simulink model "SPGF_FSK_0000_R2020b"  (R2020b)
settings: Solver=ode4  StartTime=0.0  StopTime=1.4  FixedStep=50e-6/50  RelTol=1e-3  EnableMultiTasking=on
undefined symbols (not defined in the file): D11, Delta
libraries: powerlib x2546, powerlib_meascontrol x183, simulink x24
(part 2 of 34)

== system SPGF_FSK_0000_R2020b/K4 ==
  fault : Subsystem  mask{FaultA=on, FaultB=off, FaultC=off, FaultResistance=0.0001, GroundResistance=1e-03, SnubberResistance=1e6, SnubberCapacitance=inf, TransitionTimes=[0.2 0.8], TheoryOfArc=None, ArcingVoltage=6000, TypeOfPause=None, NoiseSampleTime=0.04, NoiseSeed=23345, PulsePeriod=0.2, PulseWidth=20, PhaseDelay=0.2, SwitchTimes=[0.2 0.225 0.5 0.6], LimitArcNum=off, ArcingNumber=1, AddTimeDelay=off, TimeDelay=[0 0.1 0.2 ]}
      mask prompts: FaultA "Phase A Fault"; FaultB "Phase B Fault"; FaultC "Phase C Fault"; FaultResistance "Fault resistance Ron (ohms) :"; GroundResistance "Ground resistance Rg (ohms) :"; SnubberResistance "Snubbers resistance Rp (ohms) :"; SnubberCapacitance "Snubbers capacitance Cp (F) :"; TransitionTimes "Transition times (s) :"; TheoryOfArc "Theory of the arcing ground"; ArcingVoltage "Voltage of the arcing (V) :"; TypeOfPause "Add pause in the arcing ground"; NoiseSampleTime "Sample time of white noise (s) :"; NoiseSeed "Seed of white noise"; PulsePeriod "Period of pulses (s) :"; PulseWidth "Width of pulse (% of period) :"; PhaseDelay "Phase delay (sec) :"; SwitchTimes "Switch times (sec) [1,0,1,0...] :"; LimitArcNum "Limit number of arcing [N] :"; ArcingNumber "Number of uprising arcing"; AddTimeDelay "Add time delay :"; TimeDelay "Time delay between arc (sec) [1xN] :"
      mask init: same as SPGF_FSK_0000_R2020b/K1/fault
      settings: CloseFcn=|
      | en = get_param(gcb,'MaskEnables');
      | set_param(gcb,'MaskEnables',en)
      | clear enab en;
      settings: MoveFcn=|
      | en = get_param(gcb,'MaskEnables');
      | set_param(gcb,'MaskEnables',en)
      | clear enab en;
      mask Callback FaultA:
      | enab = get_param(gcb,'FaultA');
      | en = get_param(gcb,'MaskEnables');
      | % Set the 'MaskVisililities' property for each parameters
      | if strcmp(enab,'on')
      |     en{2}='off';
      |     en{3}='off';
      | % set_param(gcb,'MaskVisibilities',{'on','on','on','on','on','on','on','on','on','off','on','',''});
      | else
      |     en{2}='on';
      |     en{3}='on';
      | % set_param(gcb,'MaskVisibilities',{'on','on','on','on','on','on','on','on','on','on','on','',''});
      | end
      | set_param(gcb,'MaskEnables',en)
      | clear enab en;
      mask Callback FaultB:
      | enab = get_param(gcb,'FaultB');
      | en = get_param(gcb,'MaskEnables');
      | % Set the 'MaskVisililities' property for each parameters
      | if strcmp(enab,'on')
      |     en{1}='off';
      |     en{3}='off';
      | % set_param(gcb,'MaskVisibilities',{'on','on','on','on','on','on','on','on','on','off','on','',''});
      | else
      |     en{1}='on';
      |     en{3}='on';
      | % set_param(gcb,'MaskVisibilities',{'on','on','on','on','on','on','on','on','on','on','on','',''});
      | end
      | set_param(gcb,'MaskEnables',en)
      | clear enab en;
      mask Callback FaultC:
      | enab = get_param(gcb,'FaultC');
      | en = get_param(gcb,'MaskEnables');
      | % Set the 'MaskVisililities' property for each parameters
      | if strcmp(enab,'on')
      |     en{1}='off';
      |     en{2}='off';
      | % set_param(gcb,'MaskVisibilities',{'on','on','on','on','on','on','on','on','on','off','on','',''});
      | else
      |     en{1}='on';
      |     en{2}='on';
      | % set_param(gcb,'MaskVisibilities',{'on','on','on','on','on','on','on','on','on','on','on','',''});
      | end
      | set_param(gcb,'MaskEnables',en)
      | clear enab en;
      mask TypeOptions TheoryOfArc: None | Petersen | Peters & Slepian
      mask Callback TheoryOfArc:
      | enab = get_param(gcb,'TheoryOfArc');
      | en = get_param(gcb,'MaskEnables');
      | % Set the 'MaskVisililities' property for each parameters
      | if strcmp(enab,'None')
      |     en{10}='off';
      | % set_param(gcb,'MaskVisibilities',{'on','on','on','on','on','on','on','on','on','off','on','',''});
      | else
      |     en{10}='on';
      | % set_param(gcb,'MaskVisibilities',{'on','on','on','on','on','on','on','on','on','on','on','',''});
      | end
      | set_param(gcb,'MaskEnables',en)
      | clear enab en;
      mask TypeOptions TypeOfPause: None | White Noise | Pulse Generator | Time Dependent Pulses
      mask Callback TypeOfPause:
      | enab = get_param(gcb,'TypeOfPause');
      | en = get_param(gcb,'MaskVisibilities');
      | % Set the 'MaskVisibilities' property for each parameters
      | if strcmp(enab,'None')
      |     en{12} = 'off';
      |     en{13} = 'off';
      |     en{14} = 'off';
      |     en{15} = 'off';
      |     en{16} = 'off';
      |     en{17} = 'off';
      | % set_param(gcb,'MaskEnables',{'on','on','on','on','on','on','on','on','on','on','on','on','on'});
      | elseif strcmp(enab,'White Noise')
      |     en{12} = 'on';
      |     en{13} = 'on';
      |     en{14} = 'off';
      |     en{15} = 'off';
      |     en{16} = 'off';
      |     en{17} = 'off';
      | elseif strcmp(enab,'Pulse Generator')
      |     en{12} = 'off';
      |     en{13} = 'off';
      |     en{14} = 'on';
      |     en{15} = 'on';
      |     en{16} = 'on';
      |     en{17} = 'off';
      | else
      |     en{12} = 'off';
      |     en{13} = 'off';
      |     en{14} = 'off';
      |     en{15} = 'off';
      |     en{16} = 'off';
      |     en{17} = 'on';
      | % set_param(gcb,'Maskenables',{'on','on','on','on','on','on','on','on','on','on','on','off','off'});
      | end
      | set_param(gcb,'MaskVisibilities',en);
      | clear enab en;
      mask Callback LimitArcNum:
      | enab = get_param(gcb,'LimitArcNum');
      | en = get_param(gcb,'MaskVisibilities');
      | % Set the 'MaskVisibilities' property for each parameters
      | if strcmp(enab,'on')
      |     en{19} = 'on';
      |     en{20} = 'on';
      |     en{21} = 'on';
      | else
      |     en{19} = 'off';
      |     en{20} = 'off';
      |     set_param(gcb,'AddTimeDelay','off');
      |     en{21} = 'off';
      | % set_param(gcb,'Maskenables',{'on','on','on','on','on','on','on','on','on','on','on','off','off'});
      | end
      | set_param(gcb,'MaskVisibilities',en);
      | clear enab en;
      mask Callback AddTimeDelay:
      | enab = get_param(gcb,'AddTimeDelay');
      | en = get_param(gcb,'MaskVisibilities');
      | % Set the 'MaskVisibilities' property for each parameters
      | if strcmp(enab,'on')
      |     en{21} = 'on';
      | else
      |     en{21} = 'off';
      | % set_param(gcb,'Maskenables',{'on','on','on','on','on','on','on','on','on','on','on','off','off'});
      | end
      | set_param(gcb,'MaskVisibilities',en);
      | clear enab en;
      mask Display:
      | % port_label('input',1,'Iabc');
      | 
      | port_label('lconn',1,'A');
      | port_label('lconn',2,'B');
      | port_label('lconn',3,'C');
      | 
      | disp('   ПДЗ    ');
  meas : Subsystem
  A : PMIOPort  Side=Left
  B : PMIOPort  Port=2  Side=Left
  C : PMIOPort  Port=3  Side=Left
  connections:
  meas/LConn3 -- C/RConn1
  meas/LConn1 -- A/RConn1
  meas/LConn2 -- B/RConn1
  fault/LConn3 -- meas/RConn3
  fault/LConn2 -- meas/RConn2
  fault/LConn1 -- meas/RConn1

== system SPGF_FSK_0000_R2020b/K5 ==
  fault : Subsystem  mask{FaultA=off, FaultB=off, FaultC=off, FaultResistance=0.0001, GroundResistance=1e-03, SnubberResistance=1e6, SnubberCapacitance=inf, TransitionTimes=[1.2 1.8], TheoryOfArc=Peters & Slepian, ArcingVoltage=6000, TypeOfPause=None, NoiseSampleTime=0.04, NoiseSeed=23345, PulsePeriod=0.2, PulseWidth=20, PhaseDelay=0, SwitchTimes=[1 1.01 1.2 1.4], LimitArcNum=on, ArcingNumber=1, AddTimeDelay=off, TimeDelay=[0 0.1 0.2 ]}
      mask prompts: FaultA "Phase A Fault"; FaultB "Phase B Fault"; FaultC "Phase C Fault"; FaultResistance "Fault resistance Ron (ohms) :"; GroundResistance "Ground resistance Rg (ohms) :"; SnubberResistance "Snubbers resistance Rp (ohms) :"; SnubberCapacitance "Snubbers capacitance Cp (F) :"; TransitionTimes "Transition times (s) :"; TheoryOfArc "Theory of the arcing ground"; ArcingVoltage "Voltage of the arcing (V) :"; TypeOfPause "Add pause in the arcing ground"; NoiseSampleTime "Sample time of white noise (s) :"; NoiseSeed "Seed of white noise"; PulsePeriod "Period of pulses (s) :"; PulseWidth "Width of pulse (% of period) :"; PhaseDelay "Phase delay (sec) :"; SwitchTimes "Switch times (sec) [1,0,1,0...] :"; LimitArcNum "Limit number of arcing [N] :"; ArcingNumber "Number of uprising arcing"; AddTimeDelay "Add time delay :"; TimeDelay "Time delay between arc (sec) [1xN] :"
      mask init: same as SPGF_FSK_0000_R2020b/K1/fault
      settings: CloseFcn=|
      | en = get_param(gcb,'MaskEnables');
      | set_param(gcb,'MaskEnables',en)
      | clear enab en;
      settings: MoveFcn=|
      | en = get_param(gcb,'MaskEnables');
      | set_param(gcb,'MaskEnables',en)
      | clear enab en;
      mask Callback FaultA:
      | enab = get_param(gcb,'FaultA');
      | en = get_param(gcb,'MaskEnables');
      | % Set the 'MaskVisililities' property for each parameters
      | if strcmp(enab,'on')
      |     en{2}='off';
      |     en{3}='off';
      | % set_param(gcb,'MaskVisibilities',{'on','on','on','on','on','on','on','on','on','off','on','',''});
      | else
      |     en{2}='on';
      |     en{3}='on';
      | % set_param(gcb,'MaskVisibilities',{'on','on','on','on','on','on','on','on','on','on','on','',''});
      | end
      | set_param(gcb,'MaskEnables',en)
      | clear enab en;
      mask Callback FaultB:
      | enab = get_param(gcb,'FaultB');
      | en = get_param(gcb,'MaskEnables');
      | % Set the 'MaskVisililities' property for each parameters
      | if strcmp(enab,'on')
      |     en{1}='off';
      |     en{3}='off';
      | % set_param(gcb,'MaskVisibilities',{'on','on','on','on','on','on','on','on','on','off','on','',''});
      | else
      |     en{1}='on';
      |     en{3}='on';
      | % set_param(gcb,'MaskVisibilities',{'on','on','on','on','on','on','on','on','on','on','on','',''});
      | end
      | set_param(gcb,'MaskEnables',en)
      | clear enab en;
      mask Callback FaultC:
      | enab = get_param(gcb,'FaultC');
      | en = get_param(gcb,'MaskEnables');
      | % Set the 'MaskVisililities' property for each parameters
      | if strcmp(enab,'on')
      |     en{1}='off';
      |     en{2}='off';
      | % set_param(gcb,'MaskVisibilities',{'on','on','on','on','on','on','on','on','on','off','on','',''});
      | else
      |     en{1}='on';
      |     en{2}='on';
      | % set_param(gcb,'MaskVisibilities',{'on','on','on','on','on','on','on','on','on','on','on','',''});
      | end
      | set_param(gcb,'MaskEnables',en)
      | clear enab en;
      mask TypeOptions TheoryOfArc: None | Petersen | Peters & Slepian
      mask Callback TheoryOfArc:
      | enab = get_param(gcb,'TheoryOfArc');
      | en = get_param(gcb,'MaskEnables');
      | % Set the 'MaskVisililities' property for each parameters
      | if strcmp(enab,'None')
      |     en{10}='off';
      | % set_param(gcb,'MaskVisibilities',{'on','on','on','on','on','on','on','on','on','off','on','',''});
      | else
      |     en{10}='on';
      | % set_param(gcb,'MaskVisibilities',{'on','on','on','on','on','on','on','on','on','on','on','',''});
      | end
      | set_param(gcb,'MaskEnables',en)
      | clear enab en;
      mask TypeOptions TypeOfPause: None | White Noise | Pulse Generator | Time Dependent Pulses
      mask Callback TypeOfPause:
      | enab = get_param(gcb,'TypeOfPause');
      | en = get_param(gcb,'MaskVisibilities');
      | % Set the 'MaskVisibilities' property for each parameters
      | if strcmp(enab,'None')
      |     en{12} = 'off';
      |     en{13} = 'off';
      |     en{14} = 'off';
      |     en{15} = 'off';
      |     en{16} = 'off';
      |     en{17} = 'off';
      | % set_param(gcb,'MaskEnables',{'on','on','on','on','on','on','on','on','on','on','on','on','on'});
      | elseif strcmp(enab,'White Noise')
      |     en{12} = 'on';
      |     en{13} = 'on';
      |     en{14} = 'off';
      |     en{15} = 'off';
      |     en{16} = 'off';
      |     en{17} = 'off';
      | elseif strcmp(enab,'Pulse Generator')
      |     en{12} = 'off';
      |     en{13} = 'off';
      |     en{14} = 'on';
      |     en{15} = 'on';
      |     en{16} = 'on';
      |     en{17} = 'off';
      | else
      |     en{12} = 'off';
      |     en{13} = 'off';
      |     en{14} = 'off';
      |     en{15} = 'off';
      |     en{16} = 'off';
      |     en{17} = 'on';
      | % set_param(gcb,'Maskenables',{'on','on','on','on','on','on','on','on','on','on','on','off','off'});
      | end
      | set_param(gcb,'MaskVisibilities',en);
      | clear enab en;
      mask Callback LimitArcNum:
      | enab = get_param(gcb,'LimitArcNum');
      | en = get_param(gcb,'MaskVisibilities');
      | % Set the 'MaskVisibilities' property for each parameters
      | if strcmp(enab,'on')
      |     en{19} = 'on';
      |     en{20} = 'on';
      |     en{21} = 'on';
      | else
      |     en{19} = 'off';
      |     en{20} = 'off';
      |     set_param(gcb,'AddTimeDelay','off');
      |     en{21} = 'off';
      | % set_param(gcb,'Maskenables',{'on','on','on','on','on','on','on','on','on','on','on','off','off'});
      | end
      | set_param(gcb,'MaskVisibilities',en);
      | clear enab en;
      mask Callback AddTimeDelay:
      | enab = get_param(gcb,'AddTimeDelay');
      | en = get_param(gcb,'MaskVisibilities');
      | % Set the 'MaskVisibilities' property for each parameters
      | if strcmp(enab,'on')
      |     en{21} = 'on';
      | else
      |     en{21} = 'off';
      | % set_param(gcb,'Maskenables',{'on','on','on','on','on','on','on','on','on','on','on','off','off'});
      | end
      | set_param(gcb,'MaskVisibilities',en);
      | clear enab en;
      mask Display:
      | % port_label('input',1,'Iabc');
      | 
      | port_label('lconn',1,'A');
      | port_label('lconn',2,'B');
      | port_label('lconn',3,'C');
      | 
      | disp('   ПДЗ    ');
  meas : Subsystem
  A : PMIOPort  Side=Left
  B : PMIOPort  Port=2  Side=Left
  C : PMIOPort  Port=3  Side=Left
  connections:
  fault/LConn1 -- meas/RConn1
  fault/LConn2 -- meas/RConn2
  fault/LConn3 -- meas/RConn3
  meas/LConn2 -- B/RConn1
  meas/LConn1 -- A/RConn1
  meas/LConn3 -- C/RConn1

== system SPGF_FSK_0000_R2020b/K6 ==
  fault : Subsystem  mask{FaultA=on, FaultB=off, FaultC=off, FaultResistance=0.0001, GroundResistance=1e-03, SnubberResistance=1e6, SnubberCapacitance=inf, TransitionTimes=[0.2 0.8], TheoryOfArc=None, ArcingVoltage=6000, TypeOfPause=None, NoiseSampleTime=0.04, NoiseSeed=23345, PulsePeriod=0.2, PulseWidth=20, PhaseDelay=0, SwitchTimes=[1 1.01 1.2 1.4], LimitArcNum=off, ArcingNumber=1, AddTimeDelay=off, TimeDelay=[0 0.1 0.2 ]}
      mask prompts: FaultA "Phase A Fault"; FaultB "Phase B Fault"; FaultC "Phase C Fault"; FaultResistance "Fault resistance Ron (ohms) :"; GroundResistance "Ground resistance Rg (ohms) :"; SnubberResistance "Snubbers resistance Rp (ohms) :"; SnubberCapacitance "Snubbers capacitance Cp (F) :"; TransitionTimes "Transition times (s) :"; TheoryOfArc "Theory of the arcing ground"; ArcingVoltage "Voltage of the arcing (V) :"; TypeOfPause "Add pause in the arcing ground"; NoiseSampleTime "Sample time of white noise (s) :"; NoiseSeed "Seed of white noise"; PulsePeriod "Period of pulses (s) :"; PulseWidth "Width of pulse (% of period) :"; PhaseDelay "Phase delay (sec) :"; SwitchTimes "Switch times (sec) [1,0,1,0...] :"; LimitArcNum "Limit number of arcing [N] :"; ArcingNumber "Number of uprising arcing"; AddTimeDelay "Add time delay :"; TimeDelay "Time delay between arc (sec) [1xN] :"
      mask init: same as SPGF_FSK_0000_R2020b/K1/fault
      settings: CloseFcn=|
      | en = get_param(gcb,'MaskEnables');
      | set_param(gcb,'MaskEnables',en)
      | clear enab en;
      settings: MoveFcn=|
      | en = get_param(gcb,'MaskEnables');
      | set_param(gcb,'MaskEnables',en)
      | clear enab en;
      mask Callback FaultA:
      | enab = get_param(gcb,'FaultA');
      | en = get_param(gcb,'MaskEnables');
      | % Set the 'MaskVisililities' property for each parameters
      | if strcmp(enab,'on')
      |     en{2}='off';
      |     en{3}='off';
      | % set_param(gcb,'MaskVisibilities',{'on','on','on','on','on','on','on','on','on','off','on','',''});
      | else
      |     en{2}='on';
      |     en{3}='on';
      | % set_param(gcb,'MaskVisibilities',{'on','on','on','on','on','on','on','on','on','on','on','',''});
      | end
      | set_param(gcb,'MaskEnables',en)
      | clear enab en;
      mask Callback FaultB:
      | enab = get_param(gcb,'FaultB');
      | en = get_param(gcb,'MaskEnables');
      | % Set the 'MaskVisililities' property for each parameters
      | if strcmp(enab,'on')
      |     en{1}='off';
      |     en{3}='off';
      | % set_param(gcb,'MaskVisibilities',{'on','on','on','on','on','on','on','on','on','off','on','',''});
      | else
      |     en{1}='on';
      |     en{3}='on';
      | % set_param(gcb,'MaskVisibilities',{'on','on','on','on','on','on','on','on','on','on','on','',''});
      | end
      | set_param(gcb,'MaskEnables',en)
      | clear enab en;
      mask Callback FaultC:
      | enab = get_param(gcb,'FaultC');
      | en = get_param(gcb,'MaskEnables');
      | % Set the 'MaskVisililities' property for each parameters
      | if strcmp(enab,'on')
      |     en{1}='off';
      |     en{2}='off';
      | % set_param(gcb,'MaskVisibilities',{'on','on','on','on','on','on','on','on','on','off','on','',''});
      | else
      |     en{1}='on';
      |     en{2}='on';
      | % set_param(gcb,'MaskVisibilities',{'on','on','on','on','on','on','on','on','on','on','on','',''});
      | end
      | set_param(gcb,'MaskEnables',en)
      | clear enab en;
      mask TypeOptions TheoryOfArc: None | Petersen | Peters & Slepian
      mask Callback TheoryOfArc:
      | enab = get_param(gcb,'TheoryOfArc');
      | en = get_param(gcb,'MaskEnables');
      | % Set the 'MaskVisililities' property for each parameters
      | if strcmp(enab,'None')
      |     en{10}='off';
      | % set_param(gcb,'MaskVisibilities',{'on','on','on','on','on','on','on','on','on','off','on','',''});
      | else
      |     en{10}='on';
      | % set_param(gcb,'MaskVisibilities',{'on','on','on','on','on','on','on','on','on','on','on','',''});
      | end
      | set_param(gcb,'MaskEnables',en)
      | clear enab en;
      mask TypeOptions TypeOfPause: None | White Noise | Pulse Generator | Time Dependent Pulses
      mask Callback TypeOfPause:
      | enab = get_param(gcb,'TypeOfPause');
      | en = get_param(gcb,'MaskVisibilities');
      | % Set the 'MaskVisibilities' property for each parameters
      | if strcmp(enab,'None')
      |     en{12} = 'off';
      |     en{13} = 'off';
      |     en{14} = 'off';
      |     en{15} = 'off';
      |     en{16} = 'off';
      |     en{17} = 'off';
      | % set_param(gcb,'MaskEnables',{'on','on','on','on','on','on','on','on','on','on','on','on','on'});
      | elseif strcmp(enab,'White Noise')
      |     en{12} = 'on';
      |     en{13} = 'on';
      |     en{14} = 'off';
      |     en{15} = 'off';
      |     en{16} = 'off';
      |     en{17} = 'off';
      | elseif strcmp(enab,'Pulse Generator')
      |     en{12} = 'off';
      |     en{13} = 'off';
      |     en{14} = 'on';
      |     en{15} = 'on';
      |     en{16} = 'on';
      |     en{17} = 'off';
      | else
      |     en{12} = 'off';
      |     en{13} = 'off';
      |     en{14} = 'off';
      |     en{15} = 'off';
      |     en{16} = 'off';
      |     en{17} = 'on';
      | % set_param(gcb,'Maskenables',{'on','on','on','on','on','on','on','on','on','on','on','off','off'});
      | end
      | set_param(gcb,'MaskVisibilities',en);
      | clear enab en;
      mask Callback LimitArcNum:
      | enab = get_param(gcb,'LimitArcNum');
      | en = get_param(gcb,'MaskVisibilities');
      | % Set the 'MaskVisibilities' property for each parameters
      | if strcmp(enab,'on')
      |     en{19} = 'on';
      |     en{20} = 'on';
      |     en{21} = 'on';
      | else
      |     en{19} = 'off';
      |     en{20} = 'off';
      |     set_param(gcb,'AddTimeDelay','off');
      |     en{21} = 'off';
      | % set_param(gcb,'Maskenables',{'on','on','on','on','on','on','on','on','on','on','on','off','off'});
      | end
      | set_param(gcb,'MaskVisibilities',en);
      | clear enab en;
      mask Callback AddTimeDelay:
      | enab = get_param(gcb,'AddTimeDelay');
      | en = get_param(gcb,'MaskVisibilities');
      | % Set the 'MaskVisibilities' property for each parameters
      | if strcmp(enab,'on')
      |     en{21} = 'on';
      | else
      |     en{21} = 'off';
      | % set_param(gcb,'Maskenables',{'on','on','on','on','on','on','on','on','on','on','on','off','off'});
      | end
      | set_param(gcb,'MaskVisibilities',en);
      | clear enab en;
      mask Display:
      | % port_label('input',1,'Iabc');
      | 
      | port_label('lconn',1,'A');
      | port_label('lconn',2,'B');
      | port_label('lconn',3,'C');
      | 
      | disp('   ПДЗ    ');
  meas : Subsystem
  A : PMIOPort  Side=Left
  B : PMIOPort  Port=2  Side=Left
  C : PMIOPort  Port=3  Side=Left
  connections:
  fault/LConn1 -- meas/RConn1
  fault/LConn2 -- meas/RConn2
  fault/LConn3 -- meas/RConn3
  meas/LConn2 -- B/RConn1
  meas/LConn1 -- A/RConn1
  meas/LConn3 -- C/RConn1

== system SPGF_FSK_0000_R2020b/K8 ==
  fault : Subsystem  mask{FaultA=on, FaultB=off, FaultC=off, FaultResistance=0.0001, GroundResistance=1e-03, SnubberResistance=1e6, SnubberCapacitance=inf, TransitionTimes=[0.8 1.0], TheoryOfArc=Petersen, ArcingVoltage=6000, TypeOfPause=None, NoiseSampleTime=0.04, NoiseSeed=23345, PulsePeriod=0.2, PulseWidth=20, PhaseDelay=0, SwitchTimes=[1 1.01 1.2 1.4], LimitArcNum=on, ArcingNumber=2, AddTimeDelay=off, TimeDelay=[0 0.1 0.2 ]}
      mask prompts: FaultA "Phase A Fault"; FaultB "Phase B Fault"; FaultC "Phase C Fault"; FaultResistance "Fault resistance Ron (ohms) :"; GroundResistance "Ground resistance Rg (ohms) :"; SnubberResistance "Snubbers resistance Rp (ohms) :"; SnubberCapacitance "Snubbers capacitance Cp (F) :"; TransitionTimes "Transition times (s) :"; TheoryOfArc "Theory of the arcing ground"; ArcingVoltage "Voltage of the arcing (V) :"; TypeOfPause "Add pause in the arcing ground"; NoiseSampleTime "Sample time of white noise (s) :"; NoiseSeed "Seed of white noise"; PulsePeriod "Period of pulses (s) :"; PulseWidth "Width of pulse (% of period) :"; PhaseDelay "Phase delay (sec) :"; SwitchTimes "Switch times (sec) [1,0,1,0...] :"; LimitArcNum "Limit number of arcing [N] :"; ArcingNumber "Number of uprising arcing"; AddTimeDelay "Add time delay :"; TimeDelay "Time delay between arc (sec) [1xN] :"
      mask init: same as SPGF_FSK_0000_R2020b/K1/fault
      settings: CloseFcn=|
      | en = get_param(gcb,'MaskEnables');
      | set_param(gcb,'MaskEnables',en)
      | clear enab en;
      settings: MoveFcn=|
      | en = get_param(gcb,'MaskEnables');
      | set_param(gcb,'MaskEnables',en)
      | clear enab en;
      mask Callback FaultA:
      | enab = get_param(gcb,'FaultA');
      | en = get_param(gcb,'MaskEnables');
      | % Set the 'MaskVisililities' property for each parameters
      | if strcmp(enab,'on')
      |     en{2}='off';
      |     en{3}='off';
      | % set_param(gcb,'MaskVisibilities',{'on','on','on','on','on','on','on','on','on','off','on','',''});
      | else
      |     en{2}='on';
      |     en{3}='on';
      | % set_param(gcb,'MaskVisibilities',{'on','on','on','on','on','on','on','on','on','on','on','',''});
      | end
      | set_param(gcb,'MaskEnables',en)
      | clear enab en;
      mask Callback FaultB:
      | enab = get_param(gcb,'FaultB');
      | en = get_param(gcb,'MaskEnables');
      | % Set the 'MaskVisililities' property for each parameters
      | if strcmp(enab,'on')
      |     en{1}='off';
      |     en{3}='off';
      | % set_param(gcb,'MaskVisibilities',{'on','on','on','on','on','on','on','on','on','off','on','',''});
      | else
      |     en{1}='on';
      |     en{3}='on';
      | % set_param(gcb,'MaskVisibilities',{'on','on','on','on','on','on','on','on','on','on','on','',''});
      | end
      | set_param(gcb,'MaskEnables',en)
      | clear enab en;
      mask Callback FaultC:
      | enab = get_param(gcb,'FaultC');
      | en = get_param(gcb,'MaskEnables');
      | % Set the 'MaskVisililities' property for each parameters
      | if strcmp(enab,'on')
      |     en{1}='off';
      |     en{2}='off';
      | % set_param(gcb,'MaskVisibilities',{'on','on','on','on','on','on','on','on','on','off','on','',''});
      | else
      |     en{1}='on';
      |     en{2}='on';
      | % set_param(gcb,'MaskVisibilities',{'on','on','on','on','on','on','on','on','on','on','on','',''});
      | end
      | set_param(gcb,'MaskEnables',en)
      | clear enab en;
      mask TypeOptions TheoryOfArc: None | Petersen | Peters & Slepian
      mask Callback TheoryOfArc:
      | enab = get_param(gcb,'TheoryOfArc');
      | en = get_param(gcb,'MaskEnables');
      | % Set the 'MaskVisililities' property for each parameters
      | if strcmp(enab,'None')
      |     en{10}='off';
      | % set_param(gcb,'MaskVisibilities',{'on','on','on','on','on','on','on','on','on','off','on','',''});
      | else
      |     en{10}='on';
      | % set_param(gcb,'MaskVisibilities',{'on','on','on','on','on','on','on','on','on','on','on','',''});
      | end
      | set_param(gcb,'MaskEnables',en)
      | clear enab en;
      mask TypeOptions TypeOfPause: None | White Noise | Pulse Generator | Time Dependent Pulses
      mask Callback TypeOfPause:
      | enab = get_param(gcb,'TypeOfPause');
      | en = get_param(gcb,'MaskVisibilities');
      | % Set the 'MaskVisibilities' property for each parameters
      | if strcmp(enab,'None')
      |     en{12} = 'off';
      |     en{13} = 'off';
      |     en{14} = 'off';
      |     en{15} = 'off';
      |     en{16} = 'off';
      |     en{17} = 'off';
      | % set_param(gcb,'MaskEnables',{'on','on','on','on','on','on','on','on','on','on','on','on','on'});
      | elseif strcmp(enab,'White Noise')
      |     en{12} = 'on';
      |     en{13} = 'on';
      |     en{14} = 'off';
      |     en{15} = 'off';
      |     en{16} = 'off';
      |     en{17} = 'off';
      | elseif strcmp(enab,'Pulse Generator')
      |     en{12} = 'off';
      |     en{13} = 'off';
      |     en{14} = 'on';
      |     en{15} = 'on';
      |     en{16} = 'on';
      |     en{17} = 'off';
      | else
      |     en{12} = 'off';
      |     en{13} = 'off';
      |     en{14} = 'off';
      |     en{15} = 'off';
      |     en{16} = 'off';
      |     en{17} = 'on';
      | % set_param(gcb,'Maskenables',{'on','on','on','on','on','on','on','on','on','on','on','off','off'});
      | end
      | set_param(gcb,'MaskVisibilities',en);
      | clear enab en;
      mask Callback LimitArcNum:
      | enab = get_param(gcb,'LimitArcNum');
      | en = get_param(gcb,'MaskVisibilities');
      | % Set the 'MaskVisibilities' property for each parameters
      | if strcmp(enab,'on')
      |     en{19} = 'on';
      |     en{20} = 'on';
      |     en{21} = 'on';
      | else
      |     en{19} = 'off';
      |     en{20} = 'off';
      |     set_param(gcb,'AddTimeDelay','off');
      |     en{21} = 'off';
      | % set_param(gcb,'Maskenables',{'on','on','on','on','on','on','on','on','on','on','on','off','off'});
      | end
      | set_param(gcb,'MaskVisibilities',en);
      | clear enab en;
      mask Callback AddTimeDelay:
      | enab = get_param(gcb,'AddTimeDelay');
      | en = get_param(gcb,'MaskVisibilities');
      | % Set the 'MaskVisibilities' property for each parameters
      | if strcmp(enab,'on')
      |     en{21} = 'on';
      | else
      |     en{21} = 'off';
      | % set_param(gcb,'Maskenables',{'on','on','on','on','on','on','on','on','on','on','on','off','off'});
      | end
      | set_param(gcb,'MaskVisibilities',en);
      | clear enab en;
      mask Display:
      | % port_label('input',1,'Iabc');
      | 
      | port_label('lconn',1,'A');
      | port_label('lconn',2,'B');
      | port_label('lconn',3,'C');
      | 
      | disp('   ПДЗ    ');
  meas : Subsystem
  A : PMIOPort  Side=Left
  B : PMIOPort  Port=2  Side=Left
  C : PMIOPort  Port=3  Side=Left
  connections:
  fault/LConn1 -- meas/RConn1
  fault/LConn2 -- meas/RConn2
  fault/LConn3 -- meas/RConn3
  meas/LConn2 -- B/RConn1
  meas/LConn1 -- A/RConn1
  meas/LConn3 -- C/RConn1

== system SPGF_FSK_0000_R2020b/K9 ==
  fault : Subsystem  mask{FaultA=on, FaultB=off, FaultC=off, FaultResistance=0.0001, GroundResistance=1e-03, SnubberResistance=1e6, SnubberCapacitance=inf, TransitionTimes=[1.4 1.6], TheoryOfArc=Petersen, ArcingVoltage=6000, TypeOfPause=None, NoiseSampleTime=0.04, NoiseSeed=23345, PulsePeriod=0.2, PulseWidth=20, PhaseDelay=0, SwitchTimes=[1 1.01 1.2 1.4], LimitArcNum=on, ArcingNumber=2, AddTimeDelay=off, TimeDelay=[0 0.1 0.2 ]}
      mask prompts: FaultA "Phase A Fault"; FaultB "Phase B Fault"; FaultC "Phase C Fault"; FaultResistance "Fault resistance Ron (ohms) :"; GroundResistance "Ground resistance Rg (ohms) :"; SnubberResistance "Snubbers resistance Rp (ohms) :"; SnubberCapacitance "Snubbers capacitance Cp (F) :"; TransitionTimes "Transition times (s) :"; TheoryOfArc "Theory of the arcing ground"; ArcingVoltage "Voltage of the arcing (V) :"; TypeOfPause "Add pause in the arcing ground"; NoiseSampleTime "Sample time of white noise (s) :"; NoiseSeed "Seed of white noise"; PulsePeriod "Period of pulses (s) :"; PulseWidth "Width of pulse (% of period) :"; PhaseDelay "Phase delay (sec) :"; SwitchTimes "Switch times (sec) [1,0,1,0...] :"; LimitArcNum "Limit number of arcing [N] :"; ArcingNumber "Number of uprising arcing"; AddTimeDelay "Add time delay :"; TimeDelay "Time delay between arc (sec) [1xN] :"
      mask init: same as SPGF_FSK_0000_R2020b/K1/fault
      settings: CloseFcn=|
      | en = get_param(gcb,'MaskEnables');
      | set_param(gcb,'MaskEnables',en)
      | clear enab en;
      settings: MoveFcn=|
      | en = get_param(gcb,'MaskEnables');
      | set_param(gcb,'MaskEnables',en)
      | clear enab en;
      mask Callback FaultA:
      | enab = get_param(gcb,'FaultA');
      | en = get_param(gcb,'MaskEnables');
      | % Set the 'MaskVisililities' property for each parameters
      | if strcmp(enab,'on')
      |     en{2}='off';
      |     en{3}='off';
      | % set_param(gcb,'MaskVisibilities',{'on','on','on','on','on','on','on','on','on','off','on','',''});
      | else
      |     en{2}='on';
      |     en{3}='on';
      | % set_param(gcb,'MaskVisibilities',{'on','on','on','on','on','on','on','on','on','on','on','',''});
      | end
      | set_param(gcb,'MaskEnables',en)
      | clear enab en;
      mask Callback FaultB:
      | enab = get_param(gcb,'FaultB');
      | en = get_param(gcb,'MaskEnables');
      | % Set the 'MaskVisililities' property for each parameters
      | if strcmp(enab,'on')
      |     en{1}='off';
      |     en{3}='off';
      | % set_param(gcb,'MaskVisibilities',{'on','on','on','on','on','on','on','on','on','off','on','',''});
      | else
      |     en{1}='on';
      |     en{3}='on';
      | % set_param(gcb,'MaskVisibilities',{'on','on','on','on','on','on','on','on','on','on','on','',''});
      | end
      | set_param(gcb,'MaskEnables',en)
      | clear enab en;
      mask Callback FaultC:
      | enab = get_param(gcb,'FaultC');
      | en = get_param(gcb,'MaskEnables');
      | % Set the 'MaskVisililities' property for each parameters
      | if strcmp(enab,'on')
      |     en{1}='off';
      |     en{2}='off';
      | % set_param(gcb,'MaskVisibilities',{'on','on','on','on','on','on','on','on','on','off','on','',''});
      | else
      |     en{1}='on';
      |     en{2}='on';
      | % set_param(gcb,'MaskVisibilities',{'on','on','on','on','on','on','on','on','on','on','on','',''});
      | end
      | set_param(gcb,'MaskEnables',en)
      | clear enab en;
      mask TypeOptions TheoryOfArc: None | Petersen | Peters & Slepian
      mask Callback TheoryOfArc:
      | enab = get_param(gcb,'TheoryOfArc');
      | en = get_param(gcb,'MaskEnables');
      | % Set the 'MaskVisililities' property for each parameters
      | if strcmp(enab,'None')
      |     en{10}='off';
      | % set_param(gcb,'MaskVisibilities',{'on','on','on','on','on','on','on','on','on','off','on','',''});
      | else
      |     en{10}='on';
      | % set_param(gcb,'MaskVisibilities',{'on','on','on','on','on','on','on','on','on','on','on','',''});
      | end
      | set_param(gcb,'MaskEnables',en)
      | clear enab en;
      mask TypeOptions TypeOfPause: None | White Noise | Pulse Generator | Time Dependent Pulses
      mask Callback TypeOfPause:
      | enab = get_param(gcb,'TypeOfPause');
      | en = get_param(gcb,'MaskVisibilities');
      | % Set the 'MaskVisibilities' property for each parameters
      | if strcmp(enab,'None')
      |     en{12} = 'off';
      |     en{13} = 'off';
      |     en{14} = 'off';
      |     en{15} = 'off';
      |     en{16} = 'off';
      |     en{17} = 'off';
      | % set_param(gcb,'MaskEnables',{'on','on','on','on','on','on','on','on','on','on','on','on','on'});
      | elseif strcmp(enab,'White Noise')
      |     en{12} = 'on';
      |     en{13} = 'on';
      |     en{14} = 'off';
      |     en{15} = 'off';
      |     en{16} = 'off';
      |     en{17} = 'off';
      | elseif strcmp(enab,'Pulse Generator')
      |     en{12} = 'off';
      |     en{13} = 'off';
      |     en{14} = 'on';
      |     en{15} = 'on';
      |     en{16} = 'on';
      |     en{17} = 'off';
      | else
      |     en{12} = 'off';
      |     en{13} = 'off';
      |     en{14} = 'off';
      |     en{15} = 'off';
      |     en{16} = 'off';
      |     en{17} = 'on';
      | % set_param(gcb,'Maskenables',{'on','on','on','on','on','on','on','on','on','on','on','off','off'});
      | end
      | set_param(gcb,'MaskVisibilities',en);
      | clear enab en;
      mask Callback LimitArcNum:
      | enab = get_param(gcb,'LimitArcNum');
      | en = get_param(gcb,'MaskVisibilities');
      | % Set the 'MaskVisibilities' property for each parameters
      | if strcmp(enab,'on')
      |     en{19} = 'on';
      |     en{20} = 'on';
      |     en{21} = 'on';
      | else
      |     en{19} = 'off';
      |     en{20} = 'off';
      |     set_param(gcb,'AddTimeDelay','off');
      |     en{21} = 'off';
      | % set_param(gcb,'Maskenables',{'on','on','on','on','on','on','on','on','on','on','on','off','off'});
      | end
      | set_param(gcb,'MaskVisibilities',en);
      | clear enab en;
      mask Callback AddTimeDelay:
      | enab = get_param(gcb,'AddTimeDelay');
      | en = get_param(gcb,'MaskVisibilities');
      | % Set the 'MaskVisibilities' property for each parameters
      | if strcmp(enab,'on')
      |     en{21} = 'on';
      | else
      |     en{21} = 'off';
      | % set_param(gcb,'Maskenables',{'on','on','on','on','on','on','on','on','on','on','on','off','off'});
      | end
      | set_param(gcb,'MaskVisibilities',en);
      | clear enab en;
      mask Display:
      | % port_label('input',1,'Iabc');
      | 
      | port_label('lconn',1,'A');
      | port_label('lconn',2,'B');
      | port_label('lconn',3,'C');
      | 
      | disp('   ПДЗ    ');
  meas : Subsystem
  A : PMIOPort  Side=Left
  B : PMIOPort  Port=2  Side=Left
  C : PMIOPort  Port=3  Side=Left
  connections:
  meas/LConn3 -- C/RConn1
  meas/LConn1 -- A/RConn1
  meas/LConn2 -- B/RConn1
  fault/LConn3 -- meas/RConn3
  fault/LConn2 -- meas/RConn2
  fault/LConn1 -- meas/RConn1

== system SPGF_FSK_0000_R2020b/TP11 ==
  Load : powerlib/Elements/Three-Phase Parallel RLC Load  Commented=on  LConnTagsString=A|B|C  Configuration=Y (grounded)  NominalVoltage=380  Vabc=[1e3 1e3 1e3]  Vabcp=[1e3 1e3 1e3]  NominalFrequency=50  UnbalancedPower=off  ActivePower=896000/2  InductivePower=403200/2  CapacitivePower=0  Pabc=[10e3 9e3 11e3]  QLabc=[100 90 110]  QCabc=[100 90 110]  Pabcp=[10e3 9e3 11e3]  QLabcp=[100 90 110]  QCabcp=[100 90 110]  Measurements=None  LoadType=constant PQ
  Nonlinear Load : Subsystem  Commented=on
  Nonlinear Load 3ph : Subsystem
  Q : Subsystem
  T : powerlib/Elements/Three-Phase Transformer (Two Windings)  Winding1Connection=Y  Winding2Connection=Yg  CoreType=Three single-phase transformers  SetSaturation=on  Hysteresis=off  DataFile='hysteresis'  SetInitialFlux=off  Measurements=None  UNITS=pu  NominalPower=[800000, 50]  Winding1=[10250, 0.00562500, 0.03250000]  Winding2=[400.00, 0.00562500, 0.03250000]  Rm=680.851  Lm=76.9231  L0=2  Saturation=[0 0;0.01774 0.324129;0.0487637 0.61284;0.0980856 0.825118;0.2 1;0.309543 1.08024;0.652348 1.17344;2.0357 1.26115;6.0215 1.36094;12.4388 1.49469]  InitialFluxes=[-0.91260050959137 0.0304364546455671 0.882164054947387]  BreakLoop=on  DiscreteSolver=Trapezoidal iterative  DataType=off  TransfoNumber=1
  Three-Phase Series RLC Load : powerlib/Elements/Three-Phase Series RLC Load  Commented=on  LConnTagsString=A|B|C  Configuration=Y (grounded)  NominalVoltage=380  Vabc=[1e3 1e3 1e3]  Vabcp=[1e3 1e3 1e3]  NominalFrequency=50  UnbalancedPower=off  ActivePower=896000/2  InductivePower=403200/2  CapacitivePower=0  Pabc=[10e3 9e3 11e3]  QLabc=[100 90 110]  QCabc=[100 90 110]  Pabcp=[10e3 9e3 11e3]  QLabcp=[100 90 110]  QCabcp=[100 90 110]  Measurements=None  LoadType=constant Z
  Three-Phase Series RLC Load1 : powerlib/Elements/Three-Phase Series RLC Load  LConnTagsString=A|B|C  Configuration=Y (grounded)  NominalVoltage=380  Vabc=[1e3 1e3 1e3]  Vabcp=[1e3 1e3 1e3]  NominalFrequency=50  UnbalancedPower=off  ActivePower=0.1*896000/2  InductivePower=0  CapacitivePower=0  Pabc=[10e3 9e3 11e3]  QLabc=[100 90 110]  QCabc=[100 90 110]  Pabcp=[10e3 9e3 11e3]  QLabcp=[100 90 110]  QCabcp=[100 90 110]  Measurements=None  LoadType=constant Z
  Three-Phase Series RLC Load2 : powerlib/Elements/Three-Phase Series RLC Load  LConnTagsString=A|B|C  Configuration=Y (grounded)  NominalVoltage=380  Vabc=[1e3 1e3 1e3]  Vabcp=[1e3 1e3 1e3]  NominalFrequency=50  UnbalancedPower=off  ActivePower=0.9*896000/2  InductivePower=403200/2  CapacitivePower=0  Pabc=[10e3 9e3 11e3]  QLabc=[100 90 110]  QCabc=[100 90 110]  Pabcp=[10e3 9e3 11e3]  QLabcp=[100 90 110]  QCabcp=[100 90 110]  Measurements=None  LoadType=constant Z
  A : PMIOPort  Side=Right
  B : PMIOPort  Port=2  Side=Right
  C : PMIOPort  Port=3  Side=Right
  connections:
  Q/RConn2 -- B/RConn1
  Q/RConn1 -- A/RConn1
  Q/RConn3 -- C/RConn1
  Q/LConn1 -- T/LConn1
  Q/LConn2 -- T/LConn2
  Q/LConn3 -- T/LConn3
  Load/LConn2 -- Three-Phase Series RLC Load1/LConn2 -- Three-Phase Series RLC Load2/LConn2 -- Three-Phase Series RLC Load/LConn2 -- Nonlinear Load 3ph/LConn2 -- Nonlinear Load/LConn2 -- T/RConn2
  Load/LConn1 -- Three-Phase Series RLC Load1/LConn1 -- Three-Phase Series RLC Load2/LConn1 -- Three-Phase Series RLC Load/LConn1 -- Nonlinear Load 3ph/LConn1 -- Nonlinear Load/LConn1 -- T/RConn1
  Load/LConn3 -- Three-Phase Series RLC Load1/LConn3 -- Three-Phase Series RLC Load2/LConn3 -- Three-Phase Series RLC Load/LConn3 -- Nonlinear Load 3ph/LConn3 -- Nonlinear Load/LConn3 -- T/RConn3

== system SPGF_FSK_0000_R2020b/TP12 ==
  Load : powerlib/Elements/Three-Phase Parallel RLC Load  Commented=on  LConnTagsString=A|B|C  Configuration=Y (grounded)  NominalVoltage=380  Vabc=[1e3 1e3 1e3]  Vabcp=[1e3 1e3 1e3]  NominalFrequency=50  UnbalancedPower=off  ActivePower=896000  InductivePower=403200  CapacitivePower=0  Pabc=[10e3 9e3 11e3]  QLabc=[100 90 110]  QCabc=[100 90 110]  Pabcp=[10e3 9e3 11e3]  QLabcp=[100 90 110]  QCabcp=[100 90 110]  Measurements=None  LoadType=constant PQ
  Nonlinear Load : Subsystem  Commented=on
  Nonlinear Load 3ph : Subsystem
  Q : Subsystem
  T : powerlib/Elements/Three-Phase Transformer (Two Windings)  Winding1Connection=Y  Winding2Connection=Yg  CoreType=Three single-phase transformers  SetSaturation=on  Hysteresis=off  DataFile='hysteresis'  SetInitialFlux=off  Measurements=None  UNITS=pu  NominalPower=[1600000, 50]  Winding1=[10250, 0.00562500, 0.03250000]  Winding2=[400.00, 0.00562500, 0.03250000]  Rm=680.851  Lm=76.9231  L0=2  Saturation=[0 0;0.01774 0.324129;0.0487637 0.61284;0.0980856 0.825118;0.2 1;0.309543 1.08024;0.652348 1.17344;2.0357 1.26115;6.0215 1.36094;12.4388 1.49469]  InitialFluxes=[-0.906645224071723 0.0291152316046045 0.877529992467023]  BreakLoop=on  DiscreteSolver=Trapezoidal iterative  DataType=off  TransfoNumber=1
  Three-Phase Series RLC Load : powerlib/Elements/Three-Phase Series RLC Load  Commented=on  LConnTagsString=A|B|C  Configuration=Y (grounded)  NominalVoltage=380  Vabc=[1e3 1e3 1e3]  Vabcp=[1e3 1e3 1e3]  NominalFrequency=50  UnbalancedPower=off  ActivePower=896000  InductivePower=403200  CapacitivePower=0  Pabc=[10e3 9e3 11e3]  QLabc=[100 90 110]  QCabc=[100 90 110]  Pabcp=[10e3 9e3 11e3]  QLabcp=[100 90 110]  QCabcp=[100 90 110]  Measurements=None  LoadType=constant Z
  Three-Phase Series RLC Load1 : powerlib/Elements/Three-Phase Series RLC Load  LConnTagsString=A|B|C  Configuration=Y (grounded)  NominalVoltage=380  Vabc=[1e3 1e3 1e3]  Vabcp=[1e3 1e3 1e3]  NominalFrequency=50  UnbalancedPower=off  ActivePower=0.1*896000  InductivePower=0  CapacitivePower=0  Pabc=[10e3 9e3 11e3]  QLabc=[100 90 110]  QCabc=[100 90 110]  Pabcp=[10e3 9e3 11e3]  QLabcp=[100 90 110]  QCabcp=[100 90 110]  Measurements=None  LoadType=constant Z
  Three-Phase Series RLC Load2 : powerlib/Elements/Three-Phase Series RLC Load  LConnTagsString=A|B|C  Configuration=Y (grounded)  NominalVoltage=380  Vabc=[1e3 1e3 1e3]  Vabcp=[1e3 1e3 1e3]  NominalFrequency=50  UnbalancedPower=off  ActivePower=0.9*896000  InductivePower=403200  CapacitivePower=0  Pabc=[10e3 9e3 11e3]  QLabc=[100 90 110]  QCabc=[100 90 110]  Pabcp=[10e3 9e3 11e3]  QLabcp=[100 90 110]  QCabcp=[100 90 110]  Measurements=None  LoadType=constant Z
  A : PMIOPort  Side=Right
  B : PMIOPort  Port=2  Side=Right
  C : PMIOPort  Port=3  Side=Right
  connections:
  Three-Phase Series RLC Load/LConn1 -- Nonlinear Load/LConn1 -- Nonlinear Load 3ph/LConn1 -- Load/LConn1 -- T/RConn1 -- Three-Phase Series RLC Load2/LConn1 -- Three-Phase Series RLC Load1/LConn1
  Three-Phase Series RLC Load1/LConn2 -- Three-Phase Series RLC Load2/LConn2 -- Nonlinear Load/LConn2 -- Nonlinear Load 3ph/LConn2 -- T/RConn2 -- Load/LConn2 -- Three-Phase Series RLC Load/LConn2
  Three-Phase Series RLC Load1/LConn3 -- Three-Phase Series RLC Load2/LConn3 -- Nonlinear Load/LConn3 -- Nonlinear Load 3ph/LConn3 -- T/RConn3 -- Load/LConn3 -- Three-Phase Series RLC Load/LConn3
  Q/RConn3 -- C/RConn1
  Q/LConn2 -- T/LConn2
  Q/RConn1 -- A/RConn1
  Q/RConn2 -- B/RConn1
  Q/LConn1 -- T/LConn1
  Q/LConn3 -- T/LConn3

== system SPGF_FSK_0000_R2020b/TP13 ==
  Load : powerlib/Elements/Three-Phase Parallel RLC Load  Commented=on  LConnTagsString=A|B|C  Configuration=Y (grounded)  NominalVoltage=380  Vabc=[1e3 1e3 1e3]  Vabcp=[1e3 1e3 1e3]  NominalFrequency=50  UnbalancedPower=off  ActivePower=896000  InductivePower=403200  CapacitivePower=0  Pabc=[10e3 9e3 11e3]  QLabc=[100 90 110]  QCabc=[100 90 110]  Pabcp=[10e3 9e3 11e3]  QLabcp=[100 90 110]  QCabcp=[100 90 110]  Measurements=None  LoadType=constant PQ
  Nonlinear Load : Subsystem  Commented=on
  Nonlinear Load 3ph : Subsystem
  Q : Subsystem
  T : powerlib/Elements/Three-Phase Transformer (Two Windings)  Winding1Connection=Y  Winding2Connection=Yg  CoreType=Three single-phase transformers  SetSaturation=on  Hysteresis=off  DataFile='hysteresis'  SetInitialFlux=off  Measurements=None  UNITS=pu  NominalPower=[1600000, 50]  Winding1=[10250, 0.00562500, 0.03250000]  Winding2=[400.00, 0.00562500, 0.03250000]  Rm=680.851  Lm=76.9231  L0=2  Saturation=[0 0;0.01774 0.324129;0.0487637 0.61284;0.0980856 0.825118;0.2 1;0.309543 1.08024;0.652348 1.17344;2.0357 1.26115;6.0215 1.36094;12.4388 1.49469]  InitialFluxes=[-0.902496198861661 0.0282318441179589 0.874264354743799]  BreakLoop=on  DiscreteSolver=Trapezoidal iterative  DataType=off  TransfoNumber=1
  Three-Phase Series RLC Load : powerlib/Elements/Three-Phase Series RLC Load  Commented=on  LConnTagsString=A|B|C  Configuration=Y (grounded)  NominalVoltage=380  Vabc=[1e3 1e3 1e3]  Vabcp=[1e3 1e3 1e3]  NominalFrequency=50  UnbalancedPower=off  ActivePower=896000  InductivePower=403200  CapacitivePower=0  Pabc=[10e3 9e3 11e3]  QLabc=[100 90 110]  QCabc=[100 90 110]  Pabcp=[10e3 9e3 11e3]  QLabcp=[100 90 110]  QCabcp=[100 90 110]  Measurements=None  LoadType=constant Z
  Three-Phase Series RLC Load1 : powerlib/Elements/Three-Phase Series RLC Load  LConnTagsString=A|B|C  Configuration=Y (grounded)  NominalVoltage=380  Vabc=[1e3 1e3 1e3]  Vabcp=[1e3 1e3 1e3]  NominalFrequency=50  UnbalancedPower=off  ActivePower=0.1*896000  InductivePower=0  CapacitivePower=0  Pabc=[10e3 9e3 11e3]  QLabc=[100 90 110]  QCabc=[100 90 110]  Pabcp=[10e3 9e3 11e3]  QLabcp=[100 90 110]  QCabcp=[100 90 110]  Measurements=None  LoadType=constant Z
  Three-Phase Series RLC Load2 : powerlib/Elements/Three-Phase Series RLC Load  LConnTagsString=A|B|C  Configuration=Y (grounded)  NominalVoltage=380  Vabc=[1e3 1e3 1e3]  Vabcp=[1e3 1e3 1e3]  NominalFrequency=50  UnbalancedPower=off  ActivePower=0.9*896000  InductivePower=403200  CapacitivePower=0  Pabc=[10e3 9e3 11e3]  QLabc=[100 90 110]  QCabc=[100 90 110]  Pabcp=[10e3 9e3 11e3]  QLabcp=[100 90 110]  QCabcp=[100 90 110]  Measurements=None  LoadType=constant Z
  A : PMIOPort  Side=Right
  B : PMIOPort  Port=2  Side=Right
  C : PMIOPort  Port=3  Side=Right
  connections:
  Three-Phase Series RLC Load/LConn1 -- Nonlinear Load/LConn1 -- Nonlinear Load 3ph/LConn1 -- T/RConn1 -- Load/LConn1 -- Three-Phase Series RLC Load1/LConn1 -- Three-Phase Series RLC Load2/LConn1
  Three-Phase Series RLC Load2/LConn2 -- Nonlinear Load/LConn2 -- Nonlinear Load 3ph/LConn2 -- Load/LConn2 -- T/RConn2 -- Three-Phase Series RLC Load/LConn2 -- Three-Phase Series RLC Load1/LConn2
  Three-Phase Series RLC Load2/LConn3 -- Nonlinear Load/LConn3 -- Nonlinear Load 3ph/LConn3 -- Load/LConn3 -- T/RConn3 -- Three-Phase Series RLC Load/LConn3 -- Three-Phase Series RLC Load1/LConn3
  Q/RConn3 -- C/RConn1
  Q/LConn2 -- T/LConn2
  Q/RConn1 -- A/RConn1
  Q/RConn2 -- B/RConn1
  Q/LConn1 -- T/LConn1
  Q/LConn3 -- T/LConn3
